simulink model "reaction_pendulum_MPC"  (R2021b)
settings: Solver=FixedStepDiscrete  StartTime=0.0  StopTime=inf  FixedStep=h  RelTol=1e-3  EnableMultiTasking=on
PreLoadFcn:
  | warning('off','MATLAB:dispatcher:InexactMatch');
InitFcn:
  | hwinit
model workspace (MAT data in the model file):
  x_ref = [0; 0]
values from neighbouring files (symbols this model uses):
  A = [0.989609173212  0  0; 0  1  0.01; -0.000301949872013  -0.0950246262215  0.997224421049]    [MATRICES.mat]    (also in SS_11_5.mat = [0.9904  0  0; 0  1  0.01; -9e-05  -0.033262024  0.99812133]; WEAREGOINGHOMEMATRICES.mat = [0.989609173212  0  0; 0  1  0.01; 0.000423899858033  -0.095; current_SS.mat = [0.989609173212  0  0; 0  1  0.01; -9.34612180115e-05  -0.02; dynamicUpdateModel.m = [1.000494318995348 0.010001647563961 2.391143629140888e-07)
  Aineq = []    [Manual_MPC_Companion.m]    (also in Manual_MPC_Companion_THURSDAY.m)
  B = [4.20519003073 0 0]    [MATRICES.mat]    (also in SS_11_5.mat = [4.1334 0 0]; current_SS.mat; dynamicUpdateModel.m = [-1.828407620987413e-04; full_dynamics.m = dsys.B)
  bineq = []    [Manual_MPC_Companion.m]    (also in Manual_MPC_Companion_THURSDAY.m)
  C = [1 0 0; 0 1 0]    [MeasModel.m]    (also in SS_11_5.mat = [1  0  0; 0  1  0]; current_SS.mat = [1  0  0; 0  1  0]; full_dynamics.m = dsys.C; full_system_ID.m = sys_est.C)
  H = diag([kron(ones(1,Np), Q) kron(ones(1,Np), R)])    [Manual_MPC_Companion.m]    (also in Manual_MPC_Companion_THURSDAY.m = blkdiag(Qbar, Rbar))
  h = 0.01    [SS_11_5.mat]    (also in hwinit.m)
  lb = [-1e6*ones(nx_total,1); -ones(m*Np,1)]    [Manual_MPC_Companion.m]    (also in Manual_MPC_Companion_THURSDAY.m = [-1e6*ones(nx_total, 1); -ones(nu_total, 1)])
  ub = [1e6*ones(nx_total,1); ones(m*Np,1)]    [Manual_MPC_Companion.m]    (also in Manual_MPC_Companion_THURSDAY.m = [ 1e6*ones(nx_total, 1);  ones(nu_total, 1)])
undefined symbols (not defined in the file or in its folder): Discrete, Time
libraries: mpclib x1, ctrlSharedLib x1
settings Model: SimulationMode=external  ExtModeTrigDuration=100000  Creator=user  LastModifiedBy=jackh
settings SolverCC: AlgebraicLoopSolver=TrustRegion
settings DataIOCC: SaveFormat=Array  SignalLoggingSaveFormat=ModelDataLogs  SaveOutput=off  SignalLogging=off  DSMLogging=off  SaveTime=off  ReturnWorkspaceOutputs=off
settings OptimizationCC: ExpressionDepthLimit=2147483647  LifeSpan=inf
settings DebuggingCC: UnderspecifiedInitializationDetection=Classic  MergeDetectMultiDrivingBlocksExec=none  SolverPrmCheckMsg=warning  FcnCallInpInsideContextMsg=warning  StateNameClashWarn=warning  SFUnexpectedBacktrackingDiag=warning  SFNoUnconditionalDefaultTransitionDiag=warning  SFExecutionAtInitializationDiag=none  ArithmeticOperatorsInVariantConditions=warning
settings HardwareCC: ProdBitPerPointer=32  ProdBitPerSizeT=32  ProdBitPerPtrDiffT=32  ProdLargestAtomicFloat=None  ProdIntDivRoundTo=Undefined  ProdEndianess=Unspecified  ProdWordSize=32  ProdHWDeviceType=32-bit Generic
settings ModelReferenceCC: PropagateSignalLabelsOutOfModel=off
settings SFSimCC: SimUseLocalCustomCode=off  CustomCodeUndefinedFunction=UseInterfaceOnly
settings RTWCC: Description=rpend RTDAC/USB2 (Visual C/C++)  SystemTargetFile=rtcon_rpend_usb2.tlc  TemplateMakefile=rtcon_rpend_vc_usb2_x64.tmf  RTWUseLocalCustomCode=off
settings CodeAppCC: StateflowObjectComments=on
settings STFCustomTargetCC: ModelReferenceCompliant=off  CombineOutputUpdateFcns=on  MatFileLogging=on  GRTInterface=off  SystemTargetFile=rtcon_rpend_usb2.tlc
settings GRTTargetCC: TargetLangStandard=C89/C90 (ANSI)  ModelReferenceCompliant=off  ParMdlRefBuildCompliant=off  CompOptLevelCompliant=off  ConcurrentExecutionCompliant=off  CPPClassGenCompliant=off  UseToolchainInfoCompliant=off  ExtMode=on  ExtModeMexFile=rtcon_ext_comm
settings ConfigComp: CovMetricSettings=dw  CovSaveCumulativeToWorkspaceVar=on  CovSaveSingleToWorkspaceVar=on  CovExternalEMLEnable=off  CovSFcnEnable=off  CovBoundaryAbsTol=1.0e-5

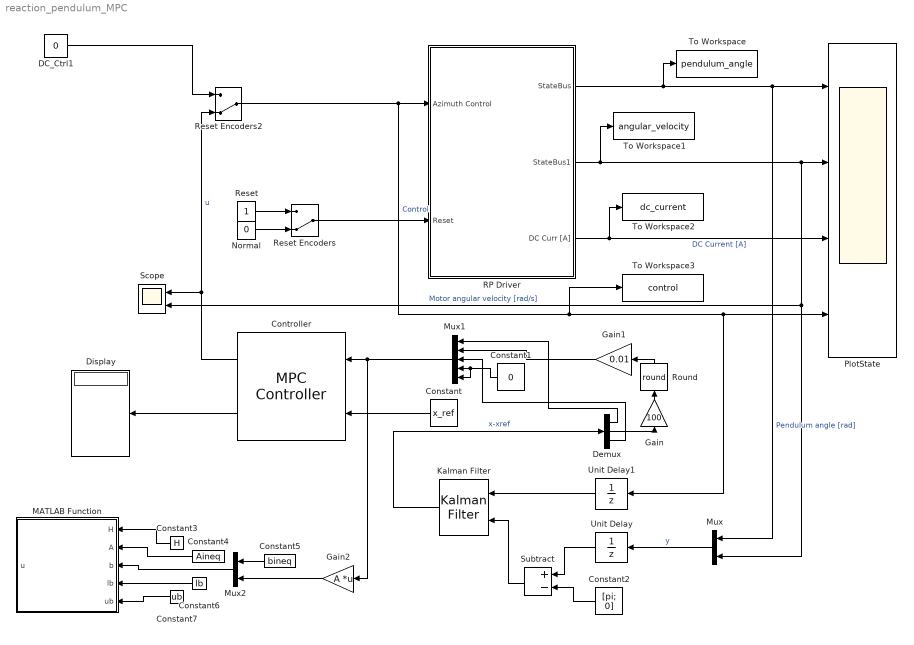
== system reaction_pendulum_MPC ==
  Constant : Constant  Value=x_ref
  Constant1 : Constant  Value=0
  Constant2 : Constant  Value=[pi; 0]
  Constant3 : Constant  Value=H
  Constant4 : Constant  Value=Aineq
  Constant5 : Constant  Value=bineq
  Constant6 : Constant  Value=lb
  Constant7 : Constant  Value=ub
  Controller : mpclib/MPC Controller  SCDEnableBlockLinearizationSpecification=on  mpcobj=MPC_controller  is_multiple=0  enable_value=0  return_u0=off  updateMPCinCallerWorkspace=on  md_inport=off  mv_inport=off  uref_inport=off  return_cost=off  return_mvseq=off  return_qpstatus=off  return_xseq=off  return_state=on  return_ovseq=off  state_inport=on  umin_inport=off  umax_inport=off  ymin_inport=off  ymax_inport=off  cc_inport=off  ywt_inport=off  uwt_inport=off  duwt_inport=off  rhoeps_inport=off  pm_inport=off  MaximumP=10  HorizonChoice=FixedHorizon  n_ts=0.01  n_p=25  n_mv=1  n_md=0  n_ud=0  n_mo=2  n_uo=0  BlockDataType=double  SampleTimeInherited=off  switch_inport=off
  DC_Ctrl1 : Constant  Value=0
  Demux : Demux  Outputs=3
  Display : Display
  Gain : Gain  Gain=100
  Gain1 : Gain  Gain=0.01
  Gain2 : Gain  Gain=A  Multiplication=Matrix(K*u) (u vector)
  Kalman Filter : ctrlSharedLib/Kalman Filter  TimeDomain=Discrete-Time  UseCurrentEstimator=on  ModelSource=Individual A, B, C, D matrices  ModelSourceVariable=ss(0.95,1,1,0,1)  A=A  B=B  C=C  D=[0;0]  NumberOfStates=1  NumberOfInputs=1  NumberOfOutputs=1  Ts=-1  InitialEstimateSource=Dialog  X0=0  P0=10  UseK=off  UseGH=off  G=1  TimeInvariantG=on  H=0  TimeInvariantH=on  NumberOfProcessNoiseInputs=1  Q=diag([0.00001 0.15 0.00001])  TimeInvariantQ=on  R=0.0001  TimeInvariantR=on  N=0  TimeInvariantN=on  AddInputPort=on  AddEnablePort=off  OutputEstimatedY=off  OutputP=off
  MATLAB Function : MATLAB Function  TreatAsAtomicUnit=on
  Mux : Mux  Inputs=2
  Mux1 : Mux  Inputs=5
  Mux2 : Mux  Inputs=2
  Normal : Constant  Value=0
  PlotState : Scope  NumInputPorts=4
  RP Driver : Subsystem
      mask Display: image(imread('rwp.JPG'))
  Reset : Constant
  Reset Encoders : ManualSwitch  CurrentSetting=0
  Reset Encoders2 : ManualSwitch  CurrentSetting=0
  Round : Rounding  Operator=round
  Scope : Scope  NumInputPorts=2
  Subtract : Sum  Inputs=+-
  To Workspace : ToWorkspace  VariableName=pendulum_angle  SaveFormat=Timeseries  SampleTime=-1
  To Workspace1 : ToWorkspace  VariableName=angular_velocity  SaveFormat=Timeseries  SampleTime=-1
  To Workspace2 : ToWorkspace  VariableName=dc_current  SaveFormat=Timeseries  SampleTime=-1
  To Workspace3 : ToWorkspace  VariableName=control  SaveFormat=Timeseries  SampleTime=-1
  Unit Delay : UnitDelay  SampleTime=h
  Unit Delay1 : UnitDelay  SampleTime=h
  wires:
  Normal/1 -> Reset Encoders/2
  Reset/1 -> Reset Encoders/1
  Reset Encoders/1 -> RP Driver/2(Reset)
  RP Driver/3(DC Curr [A]) -> To Workspace2/1, PlotState/3  "DC Current [A]"
  Reset Encoders2/1 -> Unit Delay1/1, PlotState/4, To Workspace3/1, RP Driver/1(Azimuth Control)  "Control"
  DC_Ctrl1/1 -> Reset Encoders2/1
  RP Driver/2(StateBus1) -> To Workspace1/1, Mux/2, Scope/2, PlotState/2  "Motor angular velocity [rad/s]"
  RP Driver/1(StateBus) -> Mux/1, PlotState/1, To Workspace/1  "Pendulum angle [rad]"
  Controller/1 -> Scope/1, Reset Encoders2/2  "u"
  Mux/1 -> Unit Delay/1  "y"
  Unit Delay/1 -> Subtract/1
  Controller/2 -> Display/1
  Unit Delay1/1 -> Kalman Filter/1
  Mux1/1 -> Controller/1, Gain2/1
  Constant/1 -> Controller/2
  Constant2/1 -> Subtract/2
  Subtract/1 -> Kalman Filter/2
  Kalman Filter/1 -> Demux/1  "x-xref"
  Demux/2 -> Gain/1
  Gain/1 -> Round/1
  Round/1 -> Gain1/1
  Constant1/1 -> Mux1/5, Mux1/4
  Gain1/1 -> Mux1/2
  Demux/3 -> Mux1/3
  Demux/1 -> Mux1/1
  Constant3/1 -> MATLAB Function/1(H)
  Constant7/1 -> MATLAB Function/5(ub)
  Constant6/1 -> MATLAB Function/4(lb)
  Constant4/1 -> MATLAB Function/2(A)
  Constant5/1 -> Mux2/1
  Gain2/1 -> Mux2/2
  Mux2/1 -> MATLAB Function/3(b)

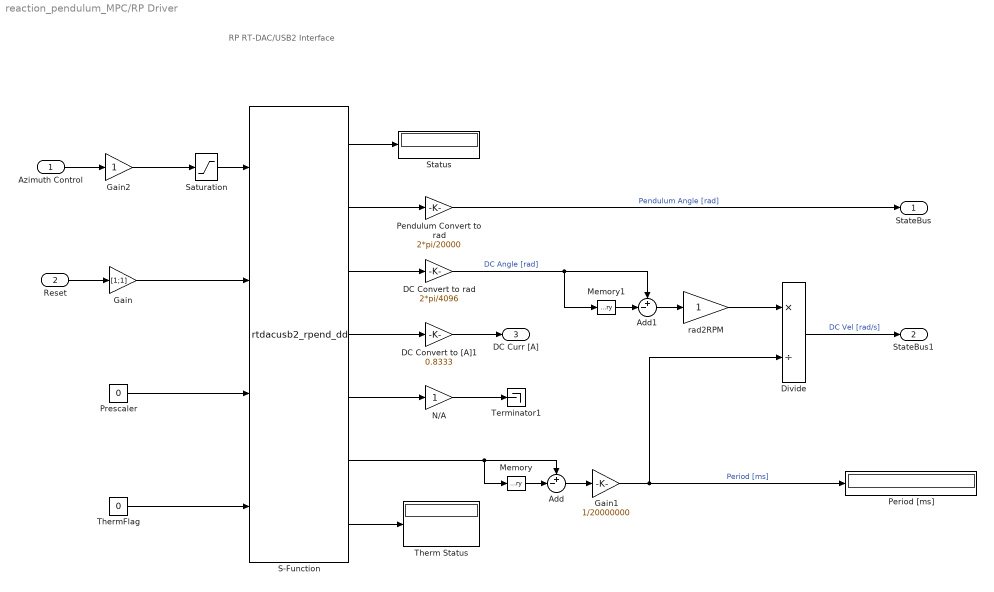
== system reaction_pendulum_MPC/RP Driver ==
  note: RP RT-DAC/USB2
      | Interface
  Azimuth Control : Inport
  Reset : Inport  Port=2
  Add : Sum  Inputs=+-|
  Add1 : Sum  Inputs=+-|
  DC Convert to [A]1 : Gain  Gain=0.8333  SaturateOnIntegerOverflow=on  OutDataTypeStr=Inherit: Same as input  ParamDataTypeStr=Inherit: Same as input
  DC Convert to rad : Gain  Gain=2*pi/4096  SaturateOnIntegerOverflow=on  OutDataTypeStr=Inherit: Same as input  ParamDataTypeStr=Inherit: Same as input
  Divide : Product  Inputs=*/
  Gain : Gain  Gain=[1;1]
  Gain1 : Gain  Gain=1/20000000
  Gain2 : Gain
  Memory : Memory
  Memory1 : Memory
  N/A : Gain  SaturateOnIntegerOverflow=on  OutDataTypeStr=Inherit: Same as input  ParamDataTypeStr=Inherit: Same as input
  Pendulum Convert to rad : Gain  Gain=2*pi/20000  SaturateOnIntegerOverflow=on  OutDataTypeStr=Inherit: Same as input  ParamDataTypeStr=Inherit: Same as input
  Period [ms] : Display
  Prescaler : Constant  Value=0
  S-Function : S-Function  FunctionName=rtdacusb2_rpend_dd  Parameters=1, h  SFunctionDeploymentMode=off  EnableBusSupport=off
  Saturation : Saturate  UpperLimit=1  LowerLimit=-1
  Status : Display
  Terminator1 : Terminator
  Therm Status : Display
  ThermFlag : Constant  Value=0
  rad2RPM : Gain  SaturateOnIntegerOverflow=on  OutDataTypeStr=Inherit: Same as input  ParamDataTypeStr=Inherit: Same as input
  StateBus : Outport  VectorParamsAs1DForOutWhenUnconnected=off
  StateBus1 : Outport  Port=2  VectorParamsAs1DForOutWhenUnconnected=off
  DC Curr [A] : Outport  Port=3  VectorParamsAs1DForOutWhenUnconnected=off
  wires:
  S-Function/7 -> Therm Status/1
  S-Function/5 -> N/A/1
  S-Function/4 -> DC Convert to [A]1/1
  ThermFlag/1 -> S-Function/4
  Prescaler/1 -> S-Function/3
  Gain/1 -> S-Function/2
  DC Convert to [A]1/1 -> DC Curr [A]/1
  Divide/1 -> StateBus1/1  "DC Vel [rad/s]"
  rad2RPM/1 -> Divide/1
  Add1/1 -> rad2RPM/1
  Memory1/1 -> Add1/2
  N/A/1 -> Terminator1/1
  S-Function/6 -> Add/1, Memory/1
  Gain2/1 -> Saturation/1
  Gain1/1 -> Period [ms]/1, Divide/2  "Period [ms]"
  Add/1 -> Gain1/1
  Memory/1 -> Add/2
  DC Convert to rad/1 -> Add1/1, Memory1/1  "DC Angle [rad]"
  S-Function/3 -> DC Convert to rad/1
  Pendulum Convert to rad/1 -> StateBus/1  "Pendulum Angle [rad]"
  S-Function/2 -> Pendulum Convert to rad/1
  S-Function/1 -> Status/1
  Saturation/1 -> S-Function/1
  Reset/1 -> Gain/1
  Azimuth Control/1 -> Gain2/1

== matlab function reaction_pendulum_MPC/MATLAB Function ==
  data: u output; H input; A input; b input; lb input; ub input
function u = MPC_short(H, A, b, lb, ub)

u = quadprog(H, [], A, b, [], [], lb, ub);
